simulink model "coolingskid_digitaltwin2"  (R2026a)
settings: Solver=VariableStepAuto  StopTime=10000
libraries: fl_lib x18, nesl_utility x10, SimscapeFluids_lib x3
settings Model: Creator=novik  LastModifiedBy=novik

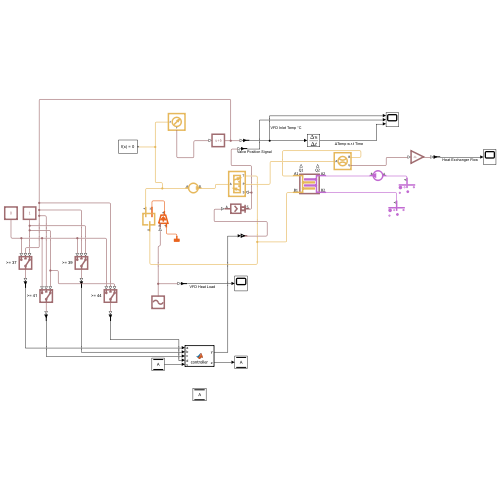
[thumbnail: Simulink's stored preview of the top-level diagram]
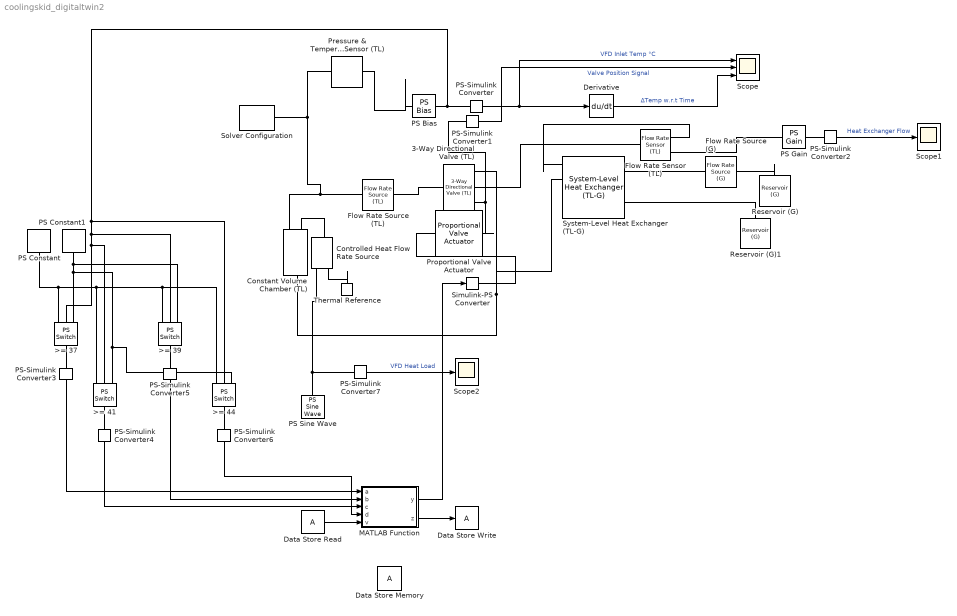
== system coolingskid_digitaltwin2 ==
  3-Way Directional Valve (TL) : SimscapeFluids_lib/Thermal Liquid/Valves & Orifices/Directional Control Valves/3-Way Directional Valve (TL)  open_orifices_pos=fluids.thermal_liquid.valves.directional_control_valves.enum.OpenOrifices3Way.PA  open_orifices_neg=fluids.thermal_liquid.valves.directional_control_valves.enum.OpenOrifices3Way.AT  area_spec=fluids.thermal_liquid.valves.directional_control_valves.enum.area_spec.identical  valve_spec=fluids.thermal_liquid.valves.directional_control_valves.enum.ValveSpec.Linear  del_S_max=5e-3 m  area_max=0.0099 m^2  del_S_TLU=[0, .00125, .0025, .00375, .005] m  valve_area_TLU=[1e-10, 1e-05, 4e-05, 8e-05, .0001] m^2  del_S_flow_TLU=[0, .00125, .0025, .00375, .005] m  p_diff_TLU=[-.1, .3, .5, .7] MPa  vol_flow_TLU=[-9.05e-10, 1.57e-09, 2.02e-09, 2.39e-09; -9.05e-05, .000157, .000202, .000239; -.000362, .000627, .00081, .000958; -.000724, .00125, .00162, .00192; -.000905, .00156, .002, .00239] m^3/s  mdot_TLU=1e3 * [-9.05e-10, 1.57e-09, 2.02e-09, 2.39e-09; -9.05e-05, .000157, .000202, .000239; -.000362, .000627, .00081, .000958; -.000724, .00125, .00162, .00192; -.000905, .00156, .002, .00239] kg/s  T_ref_in=293.15 K  p_ref_in=0.101325 MPa  area_leak=1e-10 m^2  Cd=0.64  Re_c=150  smoothing_factor=0.01  pressure_recovery=false  area=0.01 m^2  S_max_PA=2.5e-3 m  del_S_max_PA=0.005 m  area_max_PA=1e-4 m^2  del_S_TLU_PA=[0, .00125, .0025, .00375, .005] m  valve_area_TLU_PA=[1e-10, 1e-05, 4e-05, 8e-05, .0001] m^2  del_S_flow_TLU_PA=[0, .00125, .0025, .00375, .005] m  p_diff_TLU_PA=[-.1, .3, .5, .7] MPa  vol_flow_TLU_PA=[-9.05e-10, 1.57e-09, 2.02e-09, 2.39e-09; -9.05e-05, .000157, .000202, .000239; -.000362, .000627, .00081, .000958; -.000724, .00125, .00162, .00192; -.000905, .00156, .002, .00239] m^3/s  mdot_TLU_PA=1e3 * [-9.05e-10, 1.57e-09, 2.02e-09, 2.39e-09; -9.05e-05, .000157, .000202, .000239; -.000362, .000627, .00081, .000958; -.000724, .00125, .00162, .00192; -.000905, .00156, .002, .00239] kg/s  S_max_AT=-2.5e-3 m  del_S_max_AT=0.005 m  area_max_AT=1e-4 m^2  del_S_TLU_AT=[0, .00125, .0025, .00375, .005] m  valve_area_TLU_AT=[1e-10, 1e-05, 4e-05, 8e-05, .0001] m^2  del_S_flow_TLU_AT=[0, .00125, .0025, .00375, .005] m  p_diff_TLU_AT=[-.1, .3, .5, .7] MPa  vol_flow_TLU_AT=[-9.05e-10, 1.57e-09, 2.02e-09, 2.39e-09; -9.05e-05, .000157, .000202, .000239; -.000362, .000627, .00081, .000958; -.000724, .00125, .00162, .00192; -.000905, .00156, .002, .00239] m^3/s  mdot_TLU_AT=1e3 * [-9.05e-10, 1.57e-09, 2.02e-09, 2.39e-09; -9.05e-05, .000157, .000202, .000239; -.000362, .000627, .00081, .000958; -.000724, .00125, .00162, .00192; -.000905, .00156, .002, .00239] kg/s  S_max_PT=4.5e-3 m  del_S_max_PT=0.005 m  area_max_PT=1e-4 m^2  del_S_TLU_PT=[0, .00125, .0025, .00375, .005] m  valve_area_TLU_PT=[1e-10, 1e-05, 4e-05, 8e-05, .0001] m^2  del_S_flow_TLU_PT=[0, .00125, .0025, .00375, .005] m  p_diff_TLU_PT=[-.1, .3, .5, .7] MPa  vol_flow_TLU_PT=[-9.05e-10, 1.57e-09, 2.02e-09, 2.39e-09; -9.05e-05, .000157, .000202, .000239; -.000362, .000627, .00081, .000958; -.000724, .00125, .00162, .00192; -.000905, .00156, .002, .00239] m^3/s  mdot_TLU_PT=1e3 * [-9.05e-10, 1.57e-09, 2.02e-09, 2.39e-09; -9.05e-05, .000157, .000202, .000239; -.000362, .000627, .00081, .000958; -.000724, .00125, .00162, .00192; -.000905, .00156, .002, .00239] kg/s
  >= 37 : fl_lib/Physical Signals/Nonlinear Operators/PS Switch  Threshold=37 K  ZeroCross=true
  >= 39 : fl_lib/Physical Signals/Nonlinear Operators/PS Switch  Threshold=39 K  ZeroCross=true
  >= 41 : fl_lib/Physical Signals/Nonlinear Operators/PS Switch  Threshold=41 K  ZeroCross=true
  >= 44 : fl_lib/Physical Signals/Nonlinear Operators/PS Switch  Threshold=44 K  ZeroCross=true
  Constant Volume Chamber (TL) : fl_lib/Thermal Liquid/Elements/Constant Volume Chamber (TL)  volume=1 gal  num_ports=foundation.enum.num_ports.two  area_A=0.01 m^2  area_B=0.01 m^2  area_C=0.01 m^2  area_D=0.01 m^2  p_I_specify=off  p_I_priority=High  p_I=0.101325 MPa  p_I_nominal_specify=off  p_I_nominal_value=1  p_I_nominal_unit=MPa  T_I_specify=on  T_I_priority=High  T_I=25 degC  T_I_nominal_specify=off  T_I_nominal_value=1  T_I_nominal_unit=K  u_I_specify=off  u_I_priority=None  u_I=83.906 kJ/kg  u_I_nominal_specify=off  u_I_nominal_value=1  u_I_nominal_unit=kJ/kg  rho_I_specify=off  rho_I_priority=None  rho_I=998.21 kg/m^3  rho_I_nominal_specify=off  rho_I_nominal_value=1  rho_I_nominal_unit=kg/m^3
  Controlled Heat Flow Rate Source : fl_lib/Thermal/Thermal Sources/Controlled Heat Flow Rate Source
  Data Store Memory : DataStoreMemory  WriteAfterWriteMsg=warning  ShowAdditionalParam=off
  Data Store Read : DataStoreRead  IndexOptions=Index vector (dialog)  Indices=1  OutputSizes=1
  Data Store Write : DataStoreWrite  IndexOptions=Index vector (dialog)  Indices=1  OutputSizes=1
  Derivative : Derivative
  Flow Rate Sensor (TL) : fl_lib/Thermal Liquid/Sensors/Flow Rate Sensor (TL)  mass_flow_measure=false  volumetric_flow_measure=true  energy_flow_measure=false
  Flow Rate Source (TL) : fl_lib/Thermal Liquid/Sources/Flow Rate Source (TL)  source_type=foundation.enum.constant_controlled.constant  flow_type=foundation.enum.mass_volumetric_flow.volumetric  mass_flow=0 kg/s  volumetric_flow=5 gpm  power_spec=foundation.enum.power_spec.isentropic  area=0.01 m^2
  Flow Rate Source (G) : fl_lib/Gas/Sources/Flow Rate Source (G)  source_type=foundation.enum.constant_controlled.constant  flow_type=foundation.enum.mass_volumetric_flow.mass  mass_flow=4 kg/s  volumetric_flow=0 m^3/s  volumetric_flow_conditions=foundation.enum.volumetric_flow_conditions.standard  p_std=0.101325 MPa  T_std=20 degC  power_spec=foundation.enum.power_spec.isentropic  area_A=0.01 m^2  area_B=0.01 m^2
  MATLAB Function : MATLAB Function  TreatAsAtomicUnit=on
  PS Bias : fl_lib/Physical Signals/Functions/PS Bias  bias=-272.15 K
  PS Constant : fl_lib/Physical Signals/Sources/PS Constant  constant=0
  PS Constant1 : fl_lib/Physical Signals/Sources/PS Constant  constant=1
  PS Gain : fl_lib/Physical Signals/Functions/PS Gain  gain=15850.32
  PS Sine Wave : fl_lib/Physical Signals/Sources/PS Sine Wave  amplitude=600 W  bias=800 W  frequency_spec=foundation.enum.frequencySpec.frequencySI  frequency_SI=1/5000 Hz  frequency_angular=1 rad/s  phase=0 rad
  PS-Simulink Converter{,1..7} (8 alike) : nesl_utility/PS-Simulink Converter  PhysicalDomain=network_engine_domain  SubClassName=ps_output  LeftPortType=input  RightPortType=output  PseudoPeriodic=off  Frequencies=[]  VectorFormat=inherit  Unit=inherit  AffineConversion=off
  Pressure & Temperature Sensor (TL) : fl_lib/Thermal Liquid/Sensors/Pressure & Temperature Sensor (TL)  reference=foundation.enum.MeasurementReference.absolute  pressure=false  pressure_spec=foundation.enum.PressureMeasementSpec.Absolute  temperature=true
  Proportional Valve Actuator : SimscapeFluids_lib/Valve Actuators/Proportional Valve Actuator  gain=2.5e-4 m  time_constant=0.01 s  valve_stroke=0.0025 m
  Reservoir (G) : fl_lib/Gas/Elements/Reservoir (G)  pressure_input=false  pressure_spec=foundation.enum.pressure_spec.atmospheric  reservoir_pressure=0.101325 MPa  temperature_input=false  reservoir_temperature=25 degC  area_A=0.01 m^2  input_error_spec=foundation.enum.input_range_error.warn
  Reservoir (G)1 : fl_lib/Gas/Elements/Reservoir (G)  pressure_input=false  pressure_spec=foundation.enum.pressure_spec.atmospheric  reservoir_pressure=0.101325 MPa  temperature_input=false  reservoir_temperature=25 degC  area_A=0.01 m^2  input_error_spec=foundation.enum.input_range_error.warn
  Scope : Scope  NumInputPorts=3
      settings: ActiveDisplayString=3  ActiveDisplayYMinimum=-0.053541936699901933  ActiveDisplayYMaximum=0.027621642889115828  YLabel=dT/dt (°C/s)
  Scope1 : Scope
      settings: ActiveDisplayYMinimum=-0.44580028761940227  ActiveDisplayYMaximum=6.9789072431181491  YLabel=Flow Rate (gpm)
  Scope2 : Scope
      settings: ActiveDisplayYMinimum=-337.392557629099  ActiveDisplayYMaximum=1168.0845872932464  YLabel=Heat Load (W)  DataLoggingVariableName=ScopeData2
  Simulink-PS Converter : nesl_utility/Simulink-PS Converter  PhysicalDomain=network_engine_domain  SubClassName=ps_input  LeftPortType=input  RightPortType=output  PseudoPeriodic=off  Frequencies=[]  NoiseDistribution=none  NoiseParameters=[]  Unit=1  AffineConversion=off  FilteringAndDerivatives=provide  SimscapeFilterOrder=1  InputFilterTimeConstant=0.001  UdotUserProvided=0
  Solver Configuration : nesl_utility/Solver Configuration  PhysicalDomain=network_engine_domain  SubClassName=solver  LeftPortType=input  RightPortType=generic  Tones=[]  Harmonics=[]  SimulateNoise=off  Profile=off  UseLocalSampling=off  EnableSwitchedLinearOptims=on  FrequencyDomain=off  UseCCode=off  RelTol=0.001  AbsTol=0.001  MinStep=1e-09  ToWorkspace=off  RevertToSquareIcSolve=off  NumHomotopyIterations=100  PhasorMode=off  PhasorModeNumHarmonics=1  ConsistencySolver=NEWTON_XTOL_AFTER_FTOL  CanonicalOrdering=CANONICAL  OptimizeIntermediates=OPTIMIZED  IndexReductionMethod=DerivativeReplacement  DoDC=off  ResidualTolerance=1e-09  ConsistencyTolSource=GLOBAL  ConsistencyAbsTol=0.001  ConsistencyRelTol=0.001  ConsistencyTolFactor=0.001  UseLocalSolver=off  LocalSolverChoice=NE_TRAPEZOIDAL_ADVANCER  ResolveIndetEquations=on  FunctionEvalNumThread=1  LocalSolverSampleTime=0.001  DoFixedCost=off  MaxNonlinIter=3  MaxModeIter=2  ComputeImpulses=off  ImpulseIterations=2  LinearAlgebra=auto  LinearAlgebraNumThread=0  EquationFormulation=NE_TIME_EF  DelaysMemoryBudget=1024  AutomaticFiltering=on  FilteringTimeConstant=0.001  PartitionStorageMethod=AS_NEEDED  PartitionMemoryBudget=1024  PartitionMethod=FAST  MultibodyUseLocalSolver=off  MultibodyLocalSolverChoice=ODE1  MultibodyLocalSolverSampleTime=0.001
  System-Level Heat Exchanger (TL-G) : SimscapeFluids_lib/Heat Exchangers/Thermal Liquid - Gas/System-Level Heat Exchanger (TL-G)  flow_arrangement=fluids.heat_exchangers.enum.SystemLevelFlowArrangementTLG.Cross  wall_thermal_mass=false  mass_wall=1 kg  cp_wall=490 J/(K*kg)  nominal_init_wall=true  T_wall_init=293.15 K  area_A1=0.01 m^2  area_B1=0.01 m^2  area_A2=0.01 m^2  area_B2=0.01 m^2  operating_condition_TL=fluids.heat_exchangers.enum.SystemLevelOperatingConditionTLG.Cooling  mdot_nominal_TL=0.315 kg/s  delta_p_nominal_TL=0.01 MPa  p_in_nominal_TL=0.101325 MPa  T_in_nominal_TL=45 degC  capacity_spec_TL=fluids.heat_exchangers.enum.SystemLevelCapacitySpec.OutletCondition  Q_nominal=1 kW  T_out_nominal_TL=25.5 degC  volume_TL=0.001 m^3  nominal_init_TL=true  p_init_TL=0.101325 MPa  T_init_TL=293.15 K  mdot_nominal_G=4 kg/s  delta_p_nominal_G=0.001 MPa  p_in_nominal_G=0.101325 MPa  T_in_nominal_G=25 degC  volume_G=0.1 m^3  nominal_init_G=true  p_init_G=0.101325 MPa  T_init_G=293.15 K  a_TL=0.023  b_TL=0.8  c_TL=0.33  a_G=0.023  b_G=0.8  c_G=0.33
  Thermal Reference : fl_lib/Thermal/Thermal Elements/Thermal Reference
  wires:
  PS-Simulink Converter/1 -> Derivative/1, Scope/1  "VFD Inlet Temp °C"
  PS-Simulink Converter1/1 -> Scope/2  "Valve Position Signal"
  Derivative/1 -> Scope/3  "ΔTemp w.r.t Time"
  PS-Simulink Converter2/1 -> Scope1/1  "Heat Exchanger Flow"
  Data Store Read/1 -> MATLAB Function/5(v)
  MATLAB Function/2(z) -> Data Store Write/1
  PS-Simulink Converter3/1 -> MATLAB Function/1(a)
  PS-Simulink Converter4/1 -> MATLAB Function/3(c)
  PS-Simulink Converter5/1 -> MATLAB Function/2(b)
  PS-Simulink Converter6/1 -> MATLAB Function/4(d)
  MATLAB Function/1(y) -> Simulink-PS Converter/1
  PS-Simulink Converter7/1 -> Scope2/1  "VFD Heat Load"
  connections:
  Constant Volume Chamber (TL)/LConn1 -- Pressure & Temperature Sensor (TL)/LConn1 -- Solver Configuration/RConn1 -- Flow Rate Source (TL)/LConn1
  Flow Rate Source (G)/RConn1 -- System-Level Heat Exchanger (TL-G)/RConn1
  Reservoir (G)/LConn1 -- Flow Rate Source (G)/LConn1
  Reservoir (G)1/LConn1 -- System-Level Heat Exchanger (TL-G)/RConn2
  3-Way Directional Valve (TL)/LConn1 -- Flow Rate Source (TL)/RConn1
  3-Way Directional Valve (TL)/RConn3 -- System-Level Heat Exchanger (TL-G)/LConn2 -- Constant Volume Chamber (TL)/RConn1
  Pressure & Temperature Sensor (TL)/RConn1 -- PS Bias/LConn1
  PS Bias/RConn1 -- >= 44/LConn2 -- >= 41/LConn2 -- >= 37/LConn2 -- >= 39/LConn2 -- PS-Simulink Converter/LConn1
  Proportional Valve Actuator/RConn1 -- PS-Simulink Converter1/LConn1 -- 3-Way Directional Valve (TL)/RConn1
  3-Way Directional Valve (TL)/RConn2 -- Flow Rate Sensor (TL)/LConn1
  Flow Rate Sensor (TL)/RConn1 -- System-Level Heat Exchanger (TL-G)/LConn1
  Flow Rate Sensor (TL)/RConn2 -- PS Gain/LConn1
  PS-Simulink Converter2/LConn1 -- PS Gain/RConn1
  Simulink-PS Converter/RConn1 -- Proportional Valve Actuator/LConn1
  PS Constant/RConn1 -- >= 44/LConn3 -- >= 39/LConn3 -- >= 41/LConn3 -- >= 37/LConn3
  PS Constant1/RConn1 -- >= 39/LConn1 -- >= 44/LConn1 -- >= 41/LConn1 -- >= 37/LConn1
  >= 37/RConn1 -- PS-Simulink Converter3/LConn1
  PS-Simulink Converter4/LConn1 -- >= 41/RConn1
  PS-Simulink Converter5/LConn1 -- >= 39/RConn1
  PS-Simulink Converter6/LConn1 -- >= 44/RConn1
  Controlled Heat Flow Rate Source/LConn1 -- Constant Volume Chamber (TL)/LConn2
  Thermal Reference/LConn1 -- Controlled Heat Flow Rate Source/RConn2
  PS Sine Wave/RConn1 -- PS-Simulink Converter7/LConn1 -- Controlled Heat Flow Rate Source/RConn1

== matlab function coolingskid_digitaltwin2/MATLAB Function ==
  data: a input; b input; c input; d input; y output; v input; z output
function [y,z] = controller(a,b,c,d, v)
%#codegen

if a == 0
    z = 0;
    y = -10;
elseif d == 1 && (v == 2)
    z = 3;
    y = 10;
elseif c == 1 && (v == 1)
    z = 2;
    y = 5;
elseif b == 1 && (v == 0)
    z = 1;
    y = 0;
elseif a == 1 && (v == 0)
    z = 0;
    y = -10;
elseif a == 1 && (v == 1)
    z = 1;
    y = 0;
elseif a == 1 && (v == 2)
    z = 2;
    y = 5;
elseif a == 1 && (v == 3)
    z = 3;
    y = 10;
else
    z = 0;
    y = -10;
end
